simulink model "sim_anim"  (Simulink 8.2)
settings: Solver=ode45  SolverMode=SingleTasking  StartTime=0  StopTime=4  MaxStep=0.02  RelTol=1e-3  AbsTol=1e-6
values from neighbouring files (symbols this model uses):
  ref = [5 3 2]    [d_piezo.m]    (also in d_sim.m = d_sim('viewanim',sys,TR,mdl); sdt_anim.m = evalin('base','ref'); sdt_sim_anim.m = evalin('base','ref'))
undefined symbols (not defined in the file or in its folder): sdt_sim_anim
libraries: simulink x1
Description:
  | Inverted Pendulum with Animation
  | 
  | This example shows how to model an inverted pendulum.  The animation is created using MATLAB(R) Handle Graphics(R).  The animation block is a masked
  | S-function.  For more information, use the context menu to look under the Animation block's mask
  | and open the S-function for editing.
settings Model: Creator=The MathWorks Inc.  LastModifiedBy=balmes  ExtModeAutoUpdateStatusClock=off
settings DataIOCC: ExternalInput=[]  InitialState=[]  LimitDataPoints=off  SaveOutput=off  SaveTime=off
settings OptimizationCC: BlockReduction=off  BooleanDataType=off  InitFltsAndDblsToZero=on
settings DebuggingCC: SaveWithParameterizedLinksMsg=none  SignalResolutionControl=TryResolveAllWithWarning  SolverPrmCheckMsg=none  MultiTaskDSMMsg=warning  MultiTaskCondExecSysMsg=none  SigSpecEnsureSampleTimeMsg=none
settings HardwareCC: TargetUnknown=on
settings RTWCC: IncludeERTFirstTime=on
settings GRTTargetCC: TargetFcnLib=ansi_tfl_tmw.mat

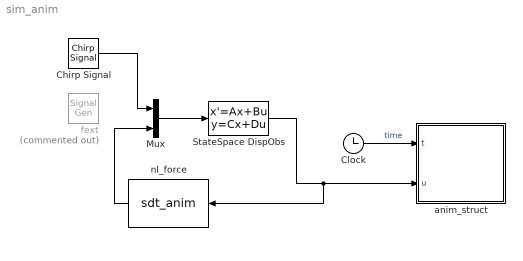
== system sim_anim ==
  Chirp Signal : simulink/Sources/Chirp Signal  f1=20  T=4  f2=200
  Clock : Clock
  Mux : Mux  Inputs=[1 2]
  StateSpace DispObs : StateSpace  A=ref.a  B=ref.b  C=ref.c  D=ref.d  X0=0  ContinuousStateAttributes='node_val'
  anim_struct : MATLAB Function  InitFcn=sdt_sim_anim('init',[]);  TreatAsAtomicUnit=on  SystemSampleTime=[0.005,0]
  fext : SignalGenerator  Commented=on  Frequency=60
  nl_force : M-S-Function  Description=Implement a non-linear force in ref.fnl  FunctionName=sdt_anim
      mask Display: disp('dt           = u(2)\ny(t + dt) = u(t)')
  wires:
  Clock/1 -> anim_struct/1(t)  "time"
  Mux/1 -> StateSpace DispObs/1
  StateSpace DispObs/1 -> nl_force/1, anim_struct/2(u)
  nl_force/1 -> Mux/2
  Chirp Signal/1 -> Mux/1

== matlab function anim_struct ==
  data: t input double; u input double
function   anim_struct(t,u)
% #codegen

coder.extrinsic('sdt_sim_anim'); % Don't compile
sdt_sim_anim(t,u);
